simulink model "car_like_system"  (R2015a)
settings: Solver=ode45  StartTime=0.0  StopTime=10.0  RelTol=1e-3
undefined symbols (not defined in the file or in its folder): InitialState
settings Model: Creator=ALVARO  LastModifiedBy=navarro
settings OptimizationCC: ExpressionDepthLimit=2147483647
settings DebuggingCC: UnderspecifiedInitializationDetection=Classic  MergeDetectMultiDrivingBlocksExec=none  SolverPrmCheckMsg=warning  StateNameClashWarn=warning

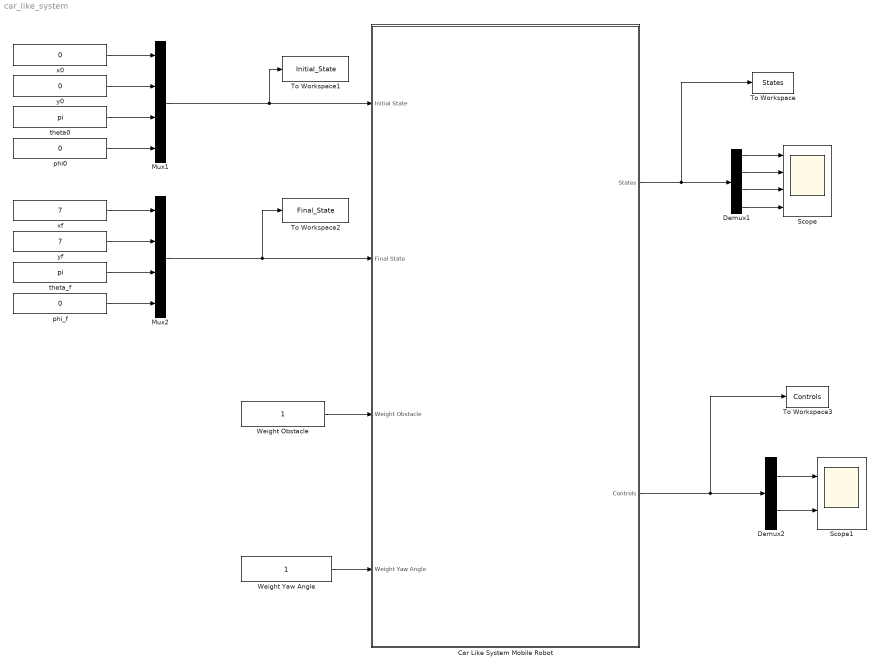
== system car_like_system ==
  Car Like System Mobile Robot : Subsystem
  Demux1 : Demux
  Demux2 : Demux  Outputs=2
  Mux1 : Mux
  Mux2 : Mux
  Scope : Scope  NumInputPorts=4
      settings: YMin=-5~-5~-5~-5  YMax=5~5~5~5
  Scope1 : Scope  NumInputPorts=2
      settings: YMin=-5~-5  YMax=5~5
  To Workspace : ToWorkspace  VariableName=States  SaveFormat=Timeseries  SampleTime=-1
  To Workspace1 : ToWorkspace  VariableName=Initial_State  SaveFormat=Timeseries  SampleTime=-1
  To Workspace2 : ToWorkspace  VariableName=Final_State  SaveFormat=Timeseries  SampleTime=-1
  To Workspace3 : ToWorkspace  VariableName=Controls  SaveFormat=Timeseries  SampleTime=-1
  Weight Obstacle : Constant
  "Weight Yaw Angle " : Constant
  phi0 : Constant  Value=0
  phi_f : Constant  Value=0
  theta0 : Constant  Value=pi
  theta_f : Constant  Value=pi
  x0 : Constant  Value=0
  xf : Constant  Value=7
  y0 : Constant  Value=0
  yf : Constant  Value=7
  wires:
  Demux1/1 -> Scope/1
  Demux1/2 -> Scope/2
  Demux1/3 -> Scope/3
  Demux1/4 -> Scope/4
  Car Like System Mobile Robot/1(States) -> Demux1/1, To Workspace/1
  "Weight Yaw Angle "/1 -> Car Like System Mobile Robot/4(Weight Yaw Angle)
  Weight Obstacle/1 -> Car Like System Mobile Robot/3(Weight Obstacle)
  x0/1 -> Mux1/1
  y0/1 -> Mux1/2
  theta0/1 -> Mux1/3
  phi0/1 -> Mux1/4
  Mux1/1 -> To Workspace1/1, Car Like System Mobile Robot/1(Initial State)
  xf/1 -> Mux2/1
  yf/1 -> Mux2/2
  theta_f/1 -> Mux2/3
  phi_f/1 -> Mux2/4
  Mux2/1 -> To Workspace2/1, Car Like System Mobile Robot/2(Final State)
  Demux2/1 -> Scope1/1
  Demux2/2 -> Scope1/2
  Car Like System Mobile Robot/2("Controls ") -> To Workspace3/1, Demux2/1

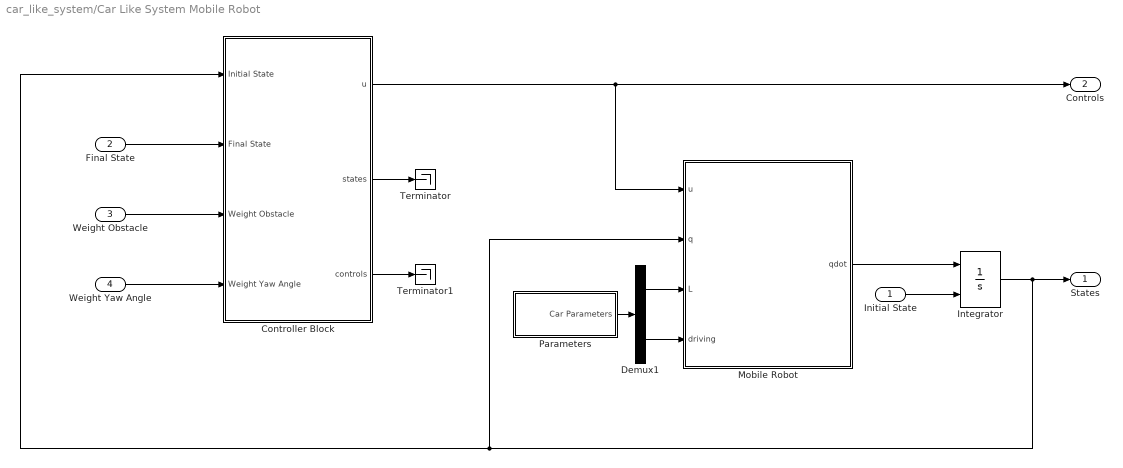
== system car_like_system/Car Like System Mobile Robot ==
  Initial State : Inport
  Final State : Inport  Port=2
  Weight Obstacle : Inport  Port=3
  Weight Yaw Angle : Inport  Port=4
  Controller Block : Subsystem
  Demux1 : Demux  Outputs=2
  Integrator : Integrator  InitialConditionSource=external  InitialCondition=InitialState
  Mobile Robot : MATLAB Function  TreatAsAtomicUnit=on
  Parameters : Subsystem
  Terminator : Terminator
  Terminator1 : Terminator
  States : Outport
  "Controls " : Outport  Port=2
  wires:
  Mobile Robot/1(qdot) -> Integrator/1
  Integrator/1 -> Controller Block/1(Initial State), Mobile Robot/2(q), States/1
  Controller Block/1(u) -> Mobile Robot/1(u), "Controls "/1
  Final State/1 -> Controller Block/2(Final State)
  Weight Yaw Angle/1 -> Controller Block/4(Weight Yaw Angle)
  Weight Obstacle/1 -> Controller Block/3(Weight Obstacle)
  Initial State/1 -> Integrator/2
  Demux1/1 -> Mobile Robot/3(L)
  Demux1/2 -> Mobile Robot/4(driving)
  Parameters/1(Car Parameters) -> Demux1/1
  Controller Block/2(states) -> Terminator/1
  Controller Block/3(controls) -> Terminator1/1

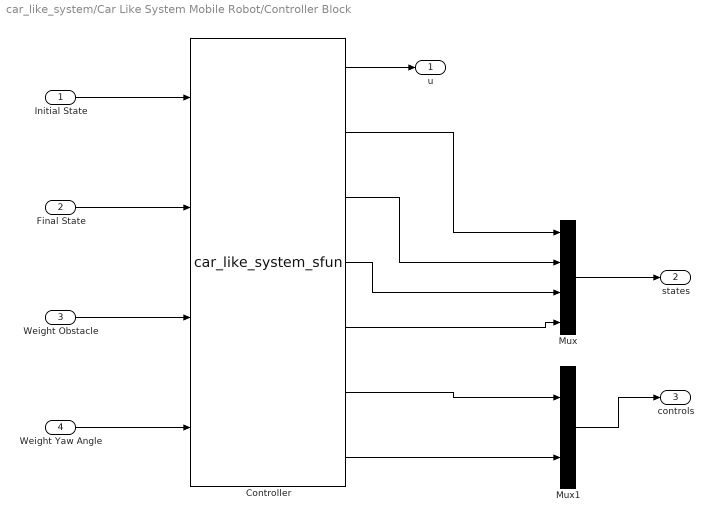
== system car_like_system/Car Like System Mobile Robot/Controller Block ==
  Initial State : Inport
  Final State : Inport  Port=2
  Weight Obstacle : Inport  Port=3
  Weight Yaw Angle : Inport  Port=4
  Controller : S-Function  FunctionName=car_like_system_sfun
  Mux : Mux
  Mux1 : Mux  Inputs=2
  u : Outport
  states : Outport  Port=2
  controls : Outport  Port=3
  wires:
  Mux/1 -> states/1
  Mux1/1 -> controls/1
  Initial State/1 -> Controller/1
  Final State/1 -> Controller/2
  Weight Obstacle/1 -> Controller/3
  Weight Yaw Angle/1 -> Controller/4
  Controller/1 -> u/1
  Controller/2 -> Mux/1
  Controller/3 -> Mux/2
  Controller/4 -> Mux/3
  Controller/5 -> Mux/4
  Controller/6 -> Mux1/1
  Controller/7 -> Mux1/2

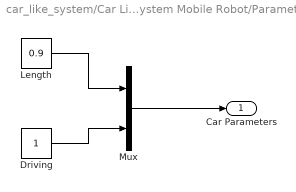
== system car_like_system/Car Like System Mobile Robot/Parameters ==
  Driving : Constant
  Length : Constant  Value=0.9
  Mux : Mux  Inputs=2
  Car Parameters : Outport
  wires:
  Mux/1 -> Car Parameters/1
  Length/1 -> Mux/1
  Driving/1 -> Mux/2

== matlab function car_like_system/Car Like System Mobile Robot/Mobile Robot ==
  data: u input; q input; qdot output; L input; driving input
function qdot = mobile_robot_car_like(u,q,L,driving)

% MOBILE_ROBOT_CAR_LIKE Computes the state space model to car like mobile
% robot taking into account where the driving is placed, either in the
% front wheels or rear wheels.
%
% The differential equations for both models are showed as follows:
%
% FRONT_WHEEL ->   
%                   qdot[0] = u[0] * Cos(x[2]) * Cos(x[3])
%                   qdot[1] = u[0] * Sin(x[2]) * Cos(x[3])
%                   qdot[2] = u[0] * Sin(x[3]) / L
%                   qdot[3] = u[1]
%
% REAR_WHEEL ->
%                   qdot[0] = u[0] * Cos(x[2])
%                   qdot[1] = u[0] * Sin(x[2])
%                   qdot[2] = u[0] * Tan(x[3]) / L
%                   qdot[3] = u[1]
% 
% Where:  qdot = (xdot, ydot, thetadot, phidot)^T and
%         q    = (x, y, theta, phi)
%         u    = (v, omega_phi)
%         L    = Length of the wheelbase
%
% Parameters
%     x              - The states (x, y, theta, phi)
%     u              - The control input (v, omega)
%     L              - Length of the wheelbase
%     driving        - This parameter identifies where the driving is
%                      placed  -> FRONT_WHEEL or REAR_WHEEL
%
% Returns
%                    The derivatives of generalized coordinates    

qdot = zeros(size(q,1),1);

if L <= 0
    disp('Invalid length of the wheelbase')
    return
end

if driving == 1
   xdot     = u(1) * cos(q(3)) * cos(q(4));
   ydot     = u(1) * sin(q(3)) * cos(q(4));
   thetadot = u(1) * sin(q(4))/L;   
else
   xdot     = u(1) * cos(q(3));
   ydot     = u(1) * sin(q(3));
   thetadot = u(1) * tan(q(4))/L;   
end

phidot = u(2);

qdot = [xdot, ydot, thetadot, phidot]';
